simulink model "BoostConverterPID_616976422"  (R2017a)
settings: Solver=VariableStepAuto  StartTime=0.0  StopTime=0.1  MaxStep=1e-4  RelTol=1e-3
undefined symbols (not defined in the file): Imag, Real
libraries: powerlib x12, simulink x2
settings Model: Creator=Weliwaththa's - ROG  LastModifiedBy=Weliwaththa's - ROG

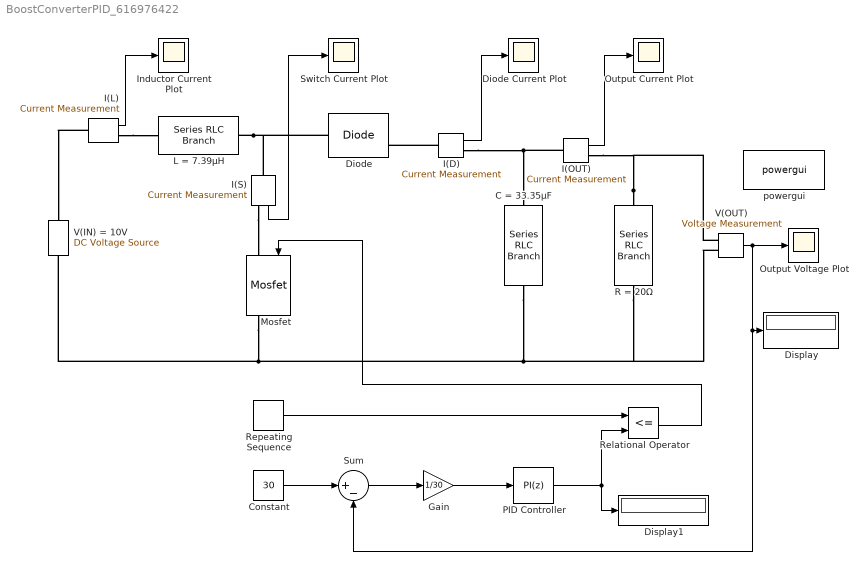
== system BoostConverterPID_616976422 ==
  C = 33.35µF : powerlib/Elements/Series RLC Branch  LConnTagsString=__new0  RConnTagsString=__new0  BranchType=C  Resistance=1  Inductance=1e-3  SetiL0=off  InitialCurrent=0  Capacitance=33.9e-6  Setx0=off  InitialVoltage=0  Measurements=None
  Constant : Constant  Value=30
  Diode : powerlib/Power Electronics/Diode  Ron=0.001  Lon=0  Vf=0.8  IC=0  UseSnubber=0  Rs=500  Cs=250e-9  Measurements=on
  Diode Current Plot : Scope
  Display : Display
  Display1 : Display
  Gain : Gain  Gain=1/30
  I(D) : powerlib/Measurements/Current Measurement  PhasorSimulation=off  OutputType=Complex  PSBequivalent=0
  I(L) : powerlib/Measurements/Current Measurement  PhasorSimulation=off  OutputType=Real-Imag  PSBequivalent=0
  I(OUT) : powerlib/Measurements/Current Measurement  PhasorSimulation=off  OutputType=Complex  PSBequivalent=0
  I(S) : powerlib/Measurements/Current Measurement  PhasorSimulation=off  OutputType=Complex  PSBequivalent=0
  Inductor Current Plot : Scope
  L = 7.39µH : powerlib/Elements/Series RLC Branch  LConnTagsString=__new0  RConnTagsString=__new0  BranchType=L  Resistance=1  Inductance=7.39e-6  SetiL0=off  InitialCurrent=0  Capacitance=1e-6  Setx0=off  InitialVoltage=0  Measurements=None
  Mosfet : powerlib/Power Electronics/Mosfet  Ron=0  Lon=0  Rd=0  Vfd=0  IC=0  Rs=1e5  Cs=inf  Measurements=on
  Output Current Plot : Scope
  Output Voltage Plot : Scope
  PID Controller : simulink/Continuous/PID Controller  Controller=PI  TimeDomain=Discrete-time  SampleTime=-1  IntegratorMethod=Forward Euler  FilterMethod=Forward Euler  Form=Parallel  UseFilter=on  ControllerParametersSource=internal  P=30  I=40.19  D=0  N=100  InitialConditionSource=internal  InitialConditionForIntegrator=0  InitialConditionForFilter=0  ExternalReset=none  LimitOutput=on  UpperSaturationLimit=0.667  LowerSaturationLimit=0.333  LinearizeAsGain=on  AntiWindupMode=none  Kb=1  TrackingMode=off  Kt=1  PParamMin=[]  PParamMax=[]  IParamMin=[]  IParamMax=[]  DParamMin=[]  DParamMax=[]  NParamMin=[]  NParamMax=[]  KbParamMin=[]  KbParamMax=[]  KtParamMin=[]  KtParamMax=[]  POutMin=[]  POutMax=[]  IOutMin=[]  IOutMax=[]  DOutMin=[]  DOutMax=[]  NOutMin=[]  NOutMax=[]  KbOutMin=[]  KbOutMax=[]  KtOutMin=[]  KtOutMax=[]  IntegratorOutMin=[]  IntegratorOutMax=[]  FilterOutMin=[]  FilterOutMax=[]  SumOutMin=[]  SumOutMax=[]  SumI1OutMin=[]  SumI1OutMax=[]  SumI2OutMin=[]  SumI2OutMax=[]  SumI3OutMin=[]  SumI3OutMax=[]  SumDOutMin=[]  SumDOutMax=[]  SaturationOutMin=[]  SaturationOutMax=[]  IntegratorContinuousStateAttributes=''  IntegratorStateMustResolveToSignalObject=off  IntegratorRTWStateStorageClass=Auto  FilterContinuousStateAttributes=''  FilterStateMustResolveToSignalObject=off  FilterRTWStateStorageClass=Auto  DifferentiatorICPrevScaledInput=0  DifferentiatorOutMin=[]  DifferentiatorOutMax=[]  InitialConditionSetting=State (most efficient)
  R = 20Ω : powerlib/Elements/Series RLC Branch  LConnTagsString=__new0  RConnTagsString=__new0  BranchType=R  Resistance=20  Inductance=1e-3  SetiL0=off  InitialCurrent=0  Capacitance=1e-6  Setx0=off  InitialVoltage=0  Measurements=None
  Relational Operator : RelationalOperator  Operator=<=  OutDataTypeStr=boolean  RndMeth=Simplest
  Repeating Sequence : simulink/Sources/Repeating Sequence  rep_seq_t=[0 0.00001]  rep_seq_y=[0 1]
  Sum : Sum  Inputs=|+-
  Switch Current Plot : Scope
  V(IN) = 10V : powerlib/Electrical Sources/DC Voltage Source  Amplitude=10  Measurements=Voltage
  V(OUT) : powerlib/Measurements/Voltage Measurement  PhasorSimulation=off  OutputType=Complex  PSBequivalent=0
  powergui : powerlib/powergui  Priority=1  SimulationMode=Continuous  SampleTime=50e-6  frequency=60  Iterations=50  frequencyindice=0  Pbase=100e6  ErrMax=1e-4  UnitsV=kV  UnitsW=MW  buscounter=0  FunctionMessages=off  echomessages=off  EnableUseOfTLC=off  CurrentSourceSwitches=off  DisableSnubberDevices=off  DisableRonSwitches=off  DisableVfSwitches=off  DisplayEquations=off  SolverType=Tustin/Backward Euler (TBE)  Interpol=off  ExternalGateDelay=off  methode=off  Ts=100  x0status=blocks  SPID=on  SwTol=0  HookPort=off  RestoreLinks=warning  ResistiveCurrentMeasurement=off  Frange=[0:2:500]  Ylog=off  Xlog=on  ShowGrid=off  save=off  variable=ZData  structure=0  ZoomFFT=off  StartTime=0.0  cycles=1  DisplayStyle=1  fundamental=60  FreqAxis=off  MaxFrequency=1000  frequencyindicesteady=1  RmsSteady=1  display=off
  wires:
  I(S)/1 -> Switch Current Plot/1
  I(OUT)/1 -> Output Current Plot/1
  I(L)/1 -> Inductor Current Plot/1
  V(OUT)/1 -> Output Voltage Plot/1, Display/1, Sum/2
  I(D)/1 -> Diode Current Plot/1
  PID Controller/1 -> Relational Operator/2, Display1/1
  Sum/1 -> Gain/1
  Constant/1 -> Sum/1
  Repeating Sequence/1 -> Relational Operator/1
  Relational Operator/1 -> Mosfet/1
  Gain/1 -> PID Controller/1
  connections:
  I(D)/RConn1 -- I(OUT)/LConn1 -- C = 33.35µF/LConn1
  V(OUT)/LConn2 -- R = 20Ω/RConn1 -- C = 33.35µF/RConn1 -- Mosfet/RConn1 -- V(IN) = 10V/LConn1
  I(L)/LConn1 -- V(IN) = 10V/RConn1
  L = 7.39µH/RConn1 -- I(S)/LConn1 -- Diode/LConn1
  R = 20Ω/LConn1 -- V(OUT)/LConn1 -- I(OUT)/RConn1
  I(D)/LConn1 -- Diode/RConn1
  I(L)/RConn1 -- L = 7.39µH/LConn1
  I(S)/RConn1 -- Mosfet/LConn1
